simulink library "HeatPump_CONF"  (R2013b)
settings: Solver=ode45  StartTime=0.0  StopTime=10.0  RelTol=1e-3
undefined symbols (not defined in the file): HP, THBout_cold, THBout_hot
libraries: carnot x3
settings Model: Creator=lena.frank  LastModifiedBy=drhf

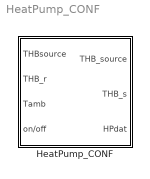
== system HeatPump_CONF ==
  HeatPump_CONF : Subsystem  mask(Heat Pump CONF){parameterfile=DefaultHeatPump}
      mask prompts: parameterfile "Parameter set"
      mask help:
      | Configurated heat pump model, variables are defined in a mat-file (for example in "DefaultHeatPump.mat"). The linearized heat pump model uses measured data (e.g. EN 14511).
      | This block uses predefined parameter sets.
      mask init:
      | % path definitions
      | intpath = fullfile(path_carnot('intlibsl'), 'Source','Heat_Pump', ...
      |     'HeatPump_CONF','parameter_set');
      | pubpath = fullfile(path_carnot('libsl'), 'Source','Heat_Pump', ...
      |     'HeatPump_CONF','parameter_set');
      | 
      | [namelist, lib] = CarnotCallbacks_getConfNamelist(intpath,pubpath);
      | 
      | if ~lib
      |     myMaskStylesVar{1} = ['popup(', namelist,')'];
      |     set_param(gcb, 'MaskStyles', myMaskStylesVar);
      | end
      | 
      | if exist(fullfile(intpath,[parameterfile '.mat']))
      |     load(fullfile(intpath,parameterfile));
      | else
      |     load(fullfile(pubpath,parameterfile));
      | end
      mask Help: web(fullfile(path_carnot('help'),'heatpump.html'),'-helpbrowser')
      mask TypeOptions parameterfile: DefaultHeatPump | Vitocal300BW_BW106 | Vitocal300BW_BW108 | Vitocal300BW_BW110 | Vitocal300BW_BW113 | Vitocal300BW_BW117
      mask Display:
      | % user defined picture file
      | picfile = fullfile(path_carnot('intlibsl'), ...
      |     'Source','Heat_Pump','HeatPump_CONF','parameter_set', ...
      |     'HeatPump_CONF.jpg');
      | 
      | pic = false;
      | 
      | % show internal picture if defined
      | if ~BlockIsInCarnotLibrary    % if not located in library any more
      |     if exist(picfile)
      |         image(imread(picfile), [0.1, 0, 0.8, 1])
      |         set_param(gcb, 'BackgroundColor', 'White')
      |         pic = true;
      |     end
      | end
      | 
      | if ~pic   % show public picture
      |     set_param(gcb, 'BackgroundColor', 'Red')
      |     plot([10,20,40,60,80,90,90,80,60,40,20,10,10]/100, ...
      |         [60,80,90,90,80,60,40,20,10,10,20,40,60]/100,[40,20]/100,...
      |         [90,20]/100,[60,80]/100,[90,20]/100,[50,50]/100, ...
      |         [30,50]/100,[60,40]/100,[40,40]/100,...
      |         [57,43]/100,[33,46]/100,[44,57]/100,[34,46]/100)
      | end
      | 
      | % Show port labels: same as port labels in the subsystem,
      | % but display with a picture covers the text. Have to reprint it.
      | port_label('input',1,'THB_source')
      | port_label('input',2,'THB_r')
      | port_label('input',3,'Tamb')
      | port_label('output',1,'THBsource')
      | port_label('output',2,'THB_s')
      | port_label('output',3,'HPdat')

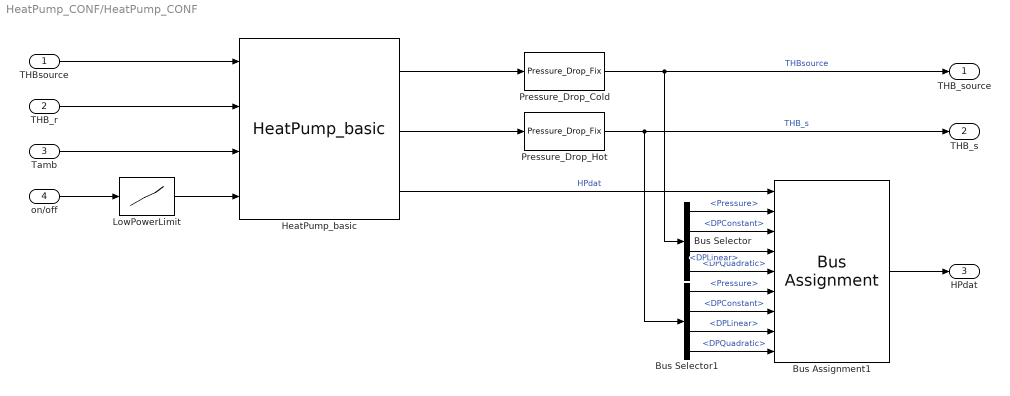
== system HeatPump_CONF/HeatPump_CONF ==
  THBsource : Inport
  THB_r : Inport  Port=2
  Tamb : Inport  Port=3
  on/off : Inport  Port=4
  Bus Assignment1 : BusAssignment  AssignedSignals=THBout_cold.Pressure,THBout_cold.DPConstant,THBout_cold.DPLinear,THBout_cold.DPQuadratic,THBout_hot.Pressure,THBout_hot.DPConstant,THBout_hot.DPLinear,THBout_hot.DPQuadratic
  Bus Selector : BusSelector  OutputSignals=Pressure,DPConstant,DPLinear,DPQuadratic
  Bus Selector1 : BusSelector  OutputSignals=Pressure,DPConstant,DPLinear,DPQuadratic
  HeatPump_basic : carnot/Basic/Thermal_Models/HeatPump_basic  K=HP.K  caph=HP.caph  capc=HP.capc  UA=HP.UA
  LowPowerLimit : Lookup  InputValues=[-1, HP.relQdotMin-eps, HP.relQdotMin, 1, 2]  Table=[0, 0, HP.relQdotMin, 1, 1]
  Pressure_Drop_Cold : carnot/Basic/Pressure_Drop/Pressure_Drop_Fix  con=0  lin=HP.linc  qua=HP.quac
  Pressure_Drop_Hot : carnot/Basic/Pressure_Drop/Pressure_Drop_Fix  con=0  lin=HP.linh  qua=HP.quah
  THB_source : Outport
  THB_s : Outport  Port=2
  HPdat : Outport  Port=3
  wires:
  Bus Selector1/4 -> Bus Assignment1/9  "<DPQuadratic>"
  Bus Selector1/3 -> Bus Assignment1/8  "<DPLinear>"
  Bus Selector1/2 -> Bus Assignment1/7  "<DPConstant>"
  Bus Selector1/1 -> Bus Assignment1/6  "<Pressure>"
  Bus Selector/4 -> Bus Assignment1/5  "<DPQuadratic>"
  Bus Selector/3 -> Bus Assignment1/4  "<DPLinear>"
  Bus Selector/2 -> Bus Assignment1/3  "<DPConstant>"
  Bus Selector/1 -> Bus Assignment1/2  "<Pressure>"
  Bus Assignment1/1 -> HPdat/1
  HeatPump_basic/3 -> Bus Assignment1/1  "HPdat"
  Pressure_Drop_Cold/1 -> Bus Selector/1, THB_source/1  "THBsource"
  HeatPump_basic/1 -> Pressure_Drop_Cold/1
  on/off/1 -> LowPowerLimit/1
  Tamb/1 -> HeatPump_basic/3
  THB_r/1 -> HeatPump_basic/2
  THBsource/1 -> HeatPump_basic/1
  HeatPump_basic/2 -> Pressure_Drop_Hot/1
  Pressure_Drop_Hot/1 -> Bus Selector1/1, THB_s/1  "THB_s"
  LowPowerLimit/1 -> HeatPump_basic/4
